simulink model "q6_2nd_order_model"  (R2024b)
settings: Solver=ode45  StartTime=0.0  StopTime=5  RelTol=1e-3
settings Model: PacingRate=0.010000  Creator=escal  LastModifiedBy=escal

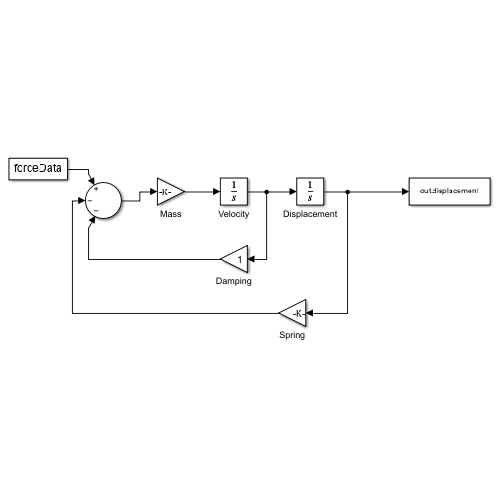
[thumbnail: Simulink's stored preview of the top-level diagram]
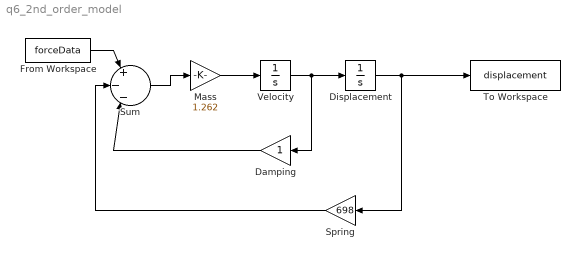
== system q6_2nd_order_model ==
  Damping : Gain
  Displacement : Integrator
  From Workspace : FromWorkspace  VariableName=forceData
  Mass : Gain  Gain=1.262
  Spring : Gain  Gain=698
  Sum : Sum  Inputs=|+|-|-|
  To Workspace : ToWorkspace  VariableName=displacement  SaveFormat=Timeseries  SampleTime=-1
  Velocity : Integrator
  wires:
  Mass/1 -> Velocity/1
  Velocity/1 -> Damping/1, Displacement/1
  Displacement/1 -> To Workspace/1, Spring/1
  Sum/1 -> Mass/1
  From Workspace/1 -> Sum/1
  Damping/1 -> Sum/3
  Spring/1 -> Sum/2
